simulink model "LMOpenLoop"  (R2014a)
settings: Solver=ode45  StartTime=0.0  StopTime=1  MaxStep=0.0034  RelTol=1e-6
settings Model: Creator=Daniel  LastModifiedBy=Daniel
settings SolverCC: ConsecutiveZCsStepRelTol=10*64*eps
settings DataIOCC: LimitDataPoints=off  Refine=20

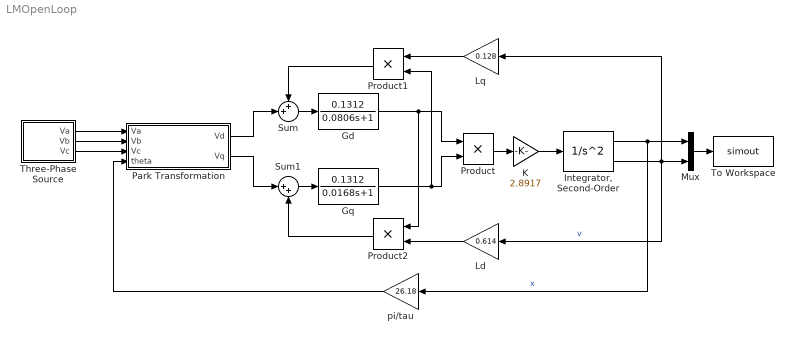
== system LMOpenLoop ==
  Gd : TransferFcn  Numerator=[0.1312]  Denominator=[0.0806 1]
  Gq : TransferFcn  Numerator=[0.1312]  Denominator=[0.0168 1]
  "Integrator, Second-Order" : SecondOrderIntegrator  ICDXDT=6.8755
  K : Gain  Gain=2.8917
  Ld : Gain  Gain=0.614
  Lq : Gain  Gain=0.128
  Mux : Mux  Inputs=2
  Park Transformation : Subsystem
  Product : Product
  Product1 : Product
  Product2 : Product
  Sum : Sum  Inputs=++|
  Sum1 : Sum  Inputs=|++
  Three-Phase Source : Subsystem
  To Workspace : ToWorkspace  VariableName=simout  SaveFormat=Timeseries  SampleTime=-1
  pi/tau : Gain  Gain=26.18
  wires:
  Three-Phase Source/1(Va) -> Park Transformation/1(Va)
  Three-Phase Source/2(Vb) -> Park Transformation/2(Vb)
  Three-Phase Source/3(Vc) -> Park Transformation/3(Vc)
  Gd/1 -> Product/1, Product2/1
  Gq/1 -> Product1/2, Product/2
  Product/1 -> K/1
  "Integrator, Second-Order"/1 -> Mux/1, pi/tau/1  "x"
  pi/tau/1 -> Park Transformation/4(theta)
  "Integrator, Second-Order"/2 -> Mux/2, Ld/1, Lq/1  "v"
  Park Transformation/1("Vd ") -> Sum/2
  Lq/1 -> Product1/1
  Product1/1 -> Sum/1
  Sum/1 -> Gd/1
  Ld/1 -> Product2/2
  Park Transformation/2(Vq) -> Sum1/1
  Product2/1 -> Sum1/2
  Sum1/1 -> Gq/1
  K/1 -> "Integrator, Second-Order"/1
  Mux/1 -> To Workspace/1

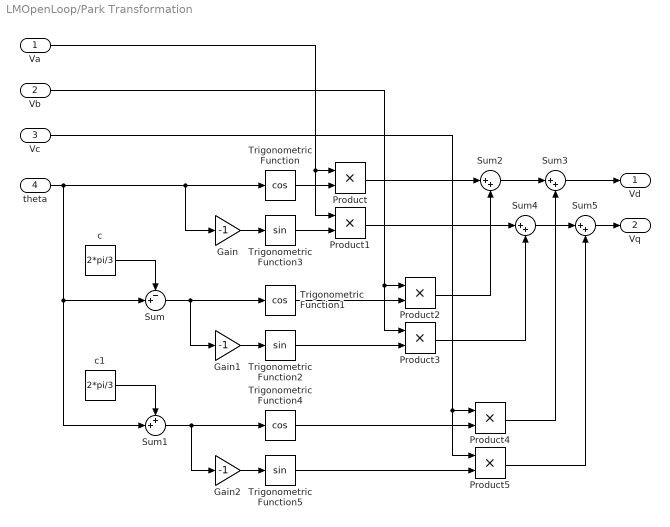
== system LMOpenLoop/Park Transformation ==
  Va : Inport
  Vb : Inport  Port=2
  Vc : Inport  Port=3
  theta : Inport  Port=4
  Gain : Gain  Gain=-1
  Gain1 : Gain  Gain=-1
  Gain2 : Gain  Gain=-1
  Product{,1..5} (6 alike) : Product
  Sum : Sum  Inputs=-+|
  Sum1 : Sum  Inputs=++|
  Sum{2..5} (4 alike) : Sum  Inputs=|++
  Trigonometric Function : Trigonometry  Operator=cos
  Trigonometric Function1 : Trigonometry  Operator=cos
  Trigonometric Function2 : Trigonometry
  Trigonometric Function3 : Trigonometry
  Trigonometric Function4 : Trigonometry  Operator=cos
  Trigonometric Function5 : Trigonometry
  c : Constant  Value=2*pi/3
  c1 : Constant  Value=2*pi/3
  "Vd " : Outport
  Vq : Outport  Port=2
  wires:
  theta/1 -> Gain/1, Trigonometric Function/1, Sum/2, Sum1/2
  c/1 -> Sum/1
  c1/1 -> Sum1/1
  Gain/1 -> Trigonometric Function3/1
  Gain1/1 -> Trigonometric Function2/1
  Gain2/1 -> Trigonometric Function5/1
  Sum/1 -> Gain1/1, Trigonometric Function1/1
  Sum1/1 -> Gain2/1, Trigonometric Function4/1
  Va/1 -> Product1/1, Product/1
  Trigonometric Function/1 -> Product/2
  Trigonometric Function3/1 -> Product1/2
  Vb/1 -> Product3/1, Product2/1
  Trigonometric Function1/1 -> Product2/2
  Trigonometric Function2/1 -> Product3/2
  Vc/1 -> Product5/1, Product4/1
  Trigonometric Function4/1 -> Product4/2
  Trigonometric Function5/1 -> Product5/2
  Product/1 -> Sum2/1
  Product2/1 -> Sum2/2
  Sum2/1 -> Sum3/1
  Product4/1 -> Sum3/2
  Product1/1 -> Sum4/1
  Product3/1 -> Sum4/2
  Sum4/1 -> Sum5/1
  Product5/1 -> Sum5/2
  Sum3/1 -> "Vd "/1
  Sum5/1 -> Vq/1

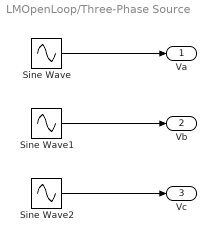
== system LMOpenLoop/Three-Phase Source ==
  Sine Wave : Sin  Amplitude=10  Frequency=180  SampleTime=0
  Sine Wave1 : Sin  Amplitude=10  Frequency=180  Phase=-2*pi/3  SampleTime=0
  Sine Wave2 : Sin  Amplitude=10  Frequency=180  Phase=2*pi/3  SampleTime=0
  Va : Outport
  Vb : Outport  Port=2
  Vc : Outport  Port=3
  wires:
  Sine Wave/1 -> Va/1
  Sine Wave1/1 -> Vb/1
  Sine Wave2/1 -> Vc/1
